simulink model "ucr_time_series_anomaly_detection_2021"  (R2021b)
settings: Solver=FixedStepDiscrete  StartTime=0.0  StopTime=100  FixedStep=0.01  RelTol=1e-3
libraries: wnnlib x38
settings Model: Creator=20214358  LastModifiedBy=20214358
settings HardwareCC: ProdLongLongMode=on  TargetBitPerPointer=64  TargetBitPerSizeT=64  TargetBitPerPtrDiffT=64  TargetLargestAtomicFloat=Float  TargetIntDivRoundTo=Zero  TargetEndianess=LittleEndian  TargetWordSize=64  TargetHWDeviceType=Intel->x86-64 (Windows64)

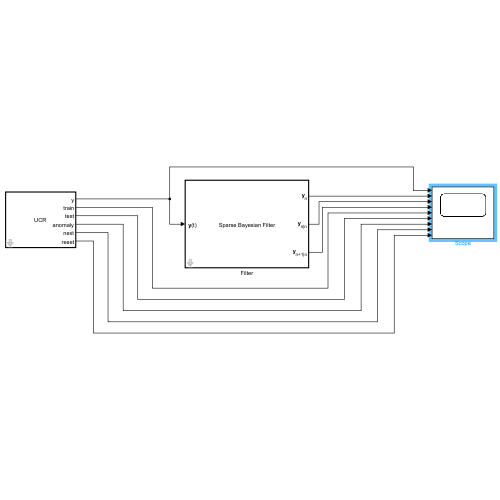
[thumbnail: Simulink's stored preview of the top-level diagram]
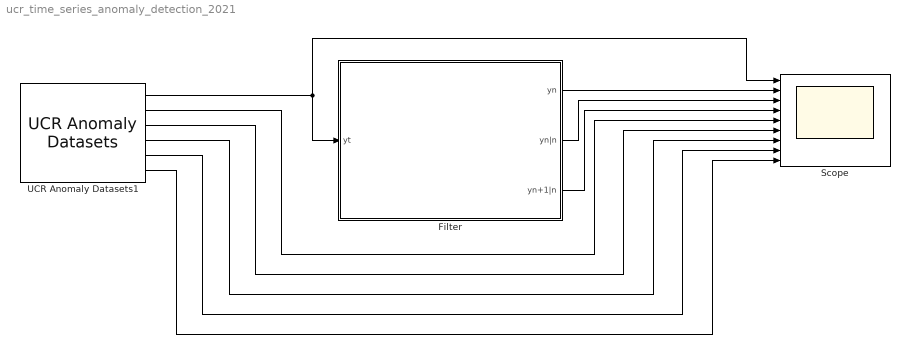
== system ucr_time_series_anomaly_detection_2021 ==
  Filter : Subsystem  TreatAsAtomicUnit=on  mask{filter_match_tolerance=1, filter_number_of_random_flips=16, sample_time=0.01, observation_dense_vector_length=1, observation_sparse_vector_length=2048, observation_memory_size=[1023 1024], observation_hamming_distance=[2 32], observation_vgram_array_length=4096, observation_number_of_samples=96, dynamics_memory_size=[1023 1024], dynamics_hamming_distance=[2 32], dynamics_vgram_array_length=2048, dynamics_number_of_samples=96, codec_number_of_sparse_vectors=4096, codec_learning_rate=0.00000000000000000000001, codec_min_bounds=[-10], codec_max_bounds=[10], codec_sparse_vectors_file='C:\Users\20214358\Workspace\wnnlib\wnndata\4k_sparse_vectors_seed_0.npz'}
      mask prompts: filter_match_tolerance "Match tolerance"; filter_number_of_random_flips "Number of random flips"; sample_time "Sample time"; observation_dense_vector_length "Dense vector length"; observation_sparse_vector_length "Sparse vector length"; observation_memory_size "Memory size"; observation_hamming_distance "Hamming distance"; observation_vgram_array_length "VGRAM array length"; observation_number_of_samples "Number of samples"; dynamics_memory_size "Memory size"; dynamics_hamming_distance "Hamming distance"; dynamics_vgram_array_length "VGRAM array length"; dynamics_number_of_samples "Number of samples"; codec_number_of_sparse_vectors "Number of sparse vectors"; codec_learning_rate "Learning rate"; codec_min_bounds "Minimum bounds"; codec_max_bounds "Maximum bounds"; codec_sparse_vectors_file "Sparse vectors file"
      mask init:
      | codec_max_kdtree_depth = ceil(log2(codec_number_of_sparse_vectors));
      | codec_min_splitting_volume = prod(codec_max_bounds - codec_min_bounds)/codec_number_of_sparse_vectors;
      | codec_sparse_vectors_file = char(codec_sparse_vectors_file);
      mask DialogControl FilterParams Prompt: Filter
      mask DialogControl ObservationModelParams Prompt: Observation model
      mask DialogControl DynamicModelParams Prompt: Dynamic model
      mask DialogControl CodecParams Prompt: Codec
      mask Display:
      | disp('Sparse Bayesian Filter','interpreter','tex');
      | port_label('input', 1,'{\bf y}(t)','interpreter','tex');
      | port_label('output', 1,'{\bf y}_{n}','interpreter','tex');
      | port_label('output', 2,'{\bf y}_{n|n}','interpreter','tex');
      | port_label('output', 3,'{\bf y}_{n+1|n}','interpreter','tex');
  Scope : Scope  NumInputPorts=9
  UCR Anomaly Datasets1 : wnnlib/Sources/UCR Anomaly Datasets  ucr_datasets_file='C:\Users\20214358\Workspace\wnnlib\wnndata\ucr_time_series_anomaly_datasets_2021.mat'  ucr_norm_flag=on  ucr_initial_dataset_idx=1  ucr_final_dataset_idx=250  ucr_sample_time=0.05
      settings: SourceProductName=Weightless Neural Networks Toolbox
  wires:
  Filter/2(yn|n) -> Scope/3
  UCR Anomaly Datasets1/1 -> Filter/1(yt), Scope/1
  Filter/1(yn) -> Scope/2
  Filter/3(yn+1|n) -> Scope/4
  UCR Anomaly Datasets1/2 -> Scope/5
  UCR Anomaly Datasets1/3 -> Scope/6
  UCR Anomaly Datasets1/4 -> Scope/7
  UCR Anomaly Datasets1/5 -> Scope/8
  UCR Anomaly Datasets1/6 -> Scope/9

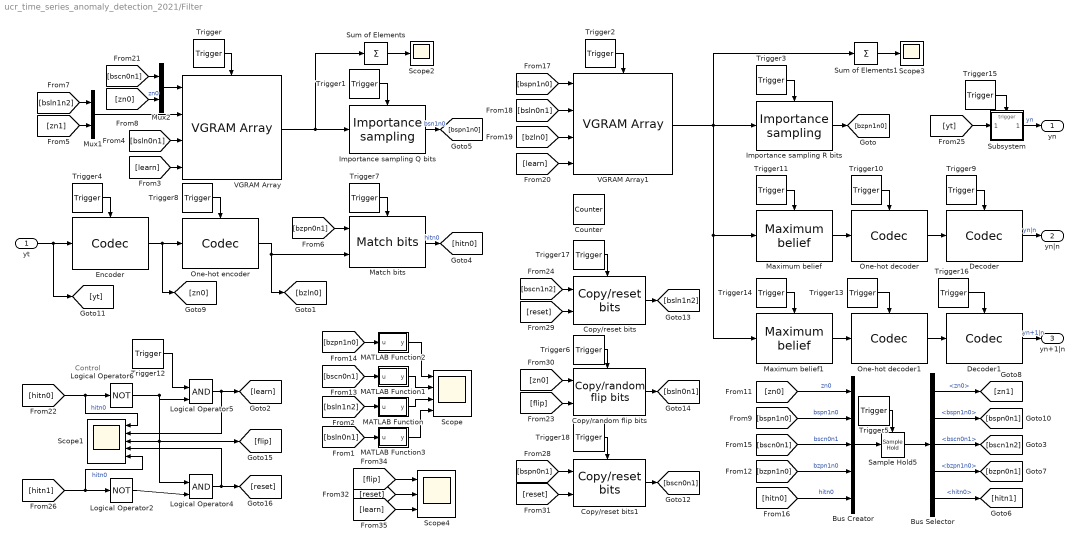
== system ucr_time_series_anomaly_detection_2021/Filter ==
  note: Control
  yt : Inport
  Bus Creator : BusCreator  Inputs=5
  Bus Selector : BusSelector  OutputSignals=zn0,bspn1n0,bscn0n1,bzpn1n0,hitn0
  Copy/random flip bits : wnnlib/Utilities/Copy//random flip bits  nNumberOfFlips=filter_number_of_random_flips
      settings: SourceProductName=Weightless Neural Networks Toolbox
  Copy/reset bits : wnnlib/Utilities/Copy//reset bits
      settings: SourceProductName=Weightless Neural Networks Toolbox
  Copy/reset bits1 : wnnlib/Utilities/Copy//reset bits
      settings: SourceProductName=Weightless Neural Networks Toolbox
  Counter : wnnlib/Sources/Counter  number_of_steps=4  sample_time=sample_time
      settings: SourceProductName=Weightless Neural Networks Toolbox
  Decoder : wnnlib/Utilities/Codec  codec_id=0  dense_vector_length=observation_dense_vector_length  sparse_vector_length=observation_sparse_vector_length  max_depth=codec_max_kdtree_depth  learning_rate=codec_learning_rate  min_splitting_volume=codec_min_splitting_volume  min_bounds=codec_min_bounds  max_bounds=codec_max_bounds  sparse_vectors_file=codec_sparse_vectors_file  debug_flag=off  codec_type=Decoder  number_of_sparse_vectors=65536
      settings: SourceProductName=Weightless Neural Networks Toolbox
  Decoder1 : wnnlib/Utilities/Codec  codec_id=0  dense_vector_length=observation_dense_vector_length  sparse_vector_length=observation_sparse_vector_length  max_depth=codec_max_kdtree_depth  learning_rate=codec_learning_rate  min_splitting_volume=codec_min_splitting_volume  min_bounds=codec_min_bounds  max_bounds=codec_max_bounds  sparse_vectors_file=codec_sparse_vectors_file  debug_flag=off  codec_type=Decoder  number_of_sparse_vectors=65536
      settings: SourceProductName=Weightless Neural Networks Toolbox
  Encoder : wnnlib/Utilities/Codec  codec_id=0  dense_vector_length=observation_dense_vector_length  sparse_vector_length=observation_sparse_vector_length  max_depth=codec_max_kdtree_depth  learning_rate=codec_learning_rate  min_splitting_volume=codec_min_splitting_volume  min_bounds=codec_min_bounds  max_bounds=codec_max_bounds  sparse_vectors_file=codec_sparse_vectors_file  debug_flag=off  codec_type=Encoder  number_of_sparse_vectors=65536
      settings: SourceProductName=Weightless Neural Networks Toolbox
  Importance sampling Q bits : wnnlib/Utilities/Importance sampling  nSamples=dynamics_number_of_samples
      settings: SourceProductName=Weightless Neural Networks Toolbox
  Importance sampling R bits : wnnlib/Utilities/Importance sampling  nSamples=observation_number_of_samples
      settings: SourceProductName=Weightless Neural Networks Toolbox
  Logical Operator2 : Logic  Operator=NOT  IconShape=distinctive  AllPortsSameDT=off  OutDataTypeStr=boolean
  Logical Operator4 : Logic  IconShape=distinctive  AllPortsSameDT=off  OutDataTypeStr=boolean
  Logical Operator5 : Logic  IconShape=distinctive  AllPortsSameDT=off  OutDataTypeStr=boolean
  Logical Operator6 : Logic  Operator=NOT  IconShape=distinctive  AllPortsSameDT=off  OutDataTypeStr=boolean
  MATLAB Function : MATLAB Function  TreatAsAtomicUnit=on
  MATLAB Function1 : MATLAB Function  TreatAsAtomicUnit=on
  MATLAB Function2 : MATLAB Function  TreatAsAtomicUnit=on
  MATLAB Function3 : MATLAB Function  TreatAsAtomicUnit=on
  Match bits : wnnlib/Utilities/Match bits  nMatchTolerance=filter_match_tolerance
      settings: SourceProductName=Weightless Neural Networks Toolbox
  Maximum belief : wnnlib/Utilities/Maximum belief  SystemSampleTime=-1  VariantActivationTime=update diagram  Latency=0  AutoFrameSizeCalculation=off
      settings: SourceProductName=Weightless Neural Networks Toolbox
  Maximum belief1 : wnnlib/Utilities/Maximum belief  SystemSampleTime=-1  VariantActivationTime=update diagram  Latency=0  AutoFrameSizeCalculation=off
      settings: SourceProductName=Weightless Neural Networks Toolbox
  Mux1 : Mux  Inputs=2
  Mux2 : Mux  Inputs=2
  One-hot decoder : wnnlib/Utilities/Codec  codec_id=0  dense_vector_length=observation_dense_vector_length  sparse_vector_length=observation_sparse_vector_length  max_depth=codec_max_kdtree_depth  learning_rate=codec_learning_rate  min_splitting_volume=codec_min_splitting_volume  min_bounds=codec_min_bounds  max_bounds=codec_max_bounds  sparse_vectors_file=codec_sparse_vectors_file  debug_flag=off  codec_type=OneHotDecoder  number_of_sparse_vectors=codec_number_of_sparse_vectors
      settings: SourceProductName=Weightless Neural Networks Toolbox
  One-hot decoder1 : wnnlib/Utilities/Codec  codec_id=0  dense_vector_length=observation_dense_vector_length  sparse_vector_length=observation_sparse_vector_length  max_depth=codec_max_kdtree_depth  learning_rate=codec_learning_rate  min_splitting_volume=codec_min_splitting_volume  min_bounds=codec_min_bounds  max_bounds=codec_max_bounds  sparse_vectors_file=codec_sparse_vectors_file  debug_flag=off  codec_type=OneHotDecoder  number_of_sparse_vectors=codec_number_of_sparse_vectors
      settings: SourceProductName=Weightless Neural Networks Toolbox
  One-hot encoder : wnnlib/Utilities/Codec  codec_id=0  dense_vector_length=observation_dense_vector_length  sparse_vector_length=observation_sparse_vector_length  max_depth=codec_max_kdtree_depth  learning_rate=codec_learning_rate  min_splitting_volume=codec_min_splitting_volume  min_bounds=codec_min_bounds  max_bounds=codec_max_bounds  sparse_vectors_file=codec_sparse_vectors_file  debug_flag=off  codec_type=OneHotEncoder  number_of_sparse_vectors=codec_number_of_sparse_vectors
      settings: SourceProductName=Weightless Neural Networks Toolbox
  Sample Hold5 : wnnlib/Utilities/Sample Hold  sample_time=-1
      settings: SourceProductName=Weightless Neural Networks Toolbox
  Scope : Scope  NumInputPorts=4
  Scope1 : Scope  NumInputPorts=5
  Scope2 : Scope
  Scope3 : Scope
  Scope4 : Scope  NumInputPorts=3
  Subsystem : Subsystem
  Sum of Elements : Sum  Inputs=+
  Sum of Elements1 : Sum  Inputs=+
  Trigger : wnnlib/Sources/Trigger  selected_steps=[0 2]
      settings: SourceProductName=Weightless Neural Networks Toolbox
  Trigger1 : wnnlib/Sources/Trigger  selected_steps=[0 2]
      settings: SourceProductName=Weightless Neural Networks Toolbox
  Trigger{4,6..12,15,17..18} (11 alike) : wnnlib/Sources/Trigger  selected_steps=0
      settings: SourceProductName=Weightless Neural Networks Toolbox
  Trigger{3,13..14,16} (4 alike) : wnnlib/Sources/Trigger  selected_steps=2
      settings: SourceProductName=Weightless Neural Networks Toolbox
  Trigger2 : wnnlib/Sources/Trigger  selected_steps=[0 2]
      settings: SourceProductName=Weightless Neural Networks Toolbox
  Trigger5 : wnnlib/Sources/Trigger  selected_steps=4
      settings: SourceProductName=Weightless Neural Networks Toolbox
  VGRAM Array : wnnlib/Models/VGRAM Array  array_id=0  min_mem_size=dynamics_memory_size(1)  max_mem_size=dynamics_memory_size(2)  min_dist=dynamics_hamming_distance(1)  max_dist=dynamics_hamming_distance(2)  pattern_length=dynamics_vgram_array_length+observation_sparse_vector_length  output_dims=[dynamics_vgram_array_length 1]  debug_flag=off
      settings: SourceProductName=Weightless Neural Networks Toolbox
  VGRAM Array1 : wnnlib/Models/VGRAM Array  array_id=1  min_mem_size=observation_memory_size(1)  max_mem_size=observation_memory_size(2)  min_dist=observation_hamming_distance(1)  max_dist=observation_hamming_distance(2)  pattern_length=dynamics_vgram_array_length  output_dims=[observation_vgram_array_length 1]  debug_flag=off
      settings: SourceProductName=Weightless Neural Networks Toolbox
  yn : Outport
  yn|n : Outport  Port=2
  yn+1|n : Outport  Port=3
  wires:
  Trigger1/1 -> Importance sampling Q bits/Trigger
  Trigger2/1 -> VGRAM Array1/Trigger
  VGRAM Array/1 -> Sum of Elements/1, Importance sampling Q bits/1
  Trigger4/1 -> Encoder/Trigger
  Trigger7/1 -> Match bits/Trigger
  Trigger6/1 -> Copy/random flip bits/Trigger
  Trigger/1 -> VGRAM Array/Trigger
  Trigger3/1 -> Importance sampling R bits/Trigger
  [bzpn0n1] -> Match bits/1
  Trigger8/1 -> One-hot encoder/Trigger
  [bsln0n1] -> VGRAM Array1/2
  Decoder/1 -> yn|n/1  "yn|n"
  Trigger9/1 -> Decoder/Trigger
  One-hot decoder/1 -> Decoder/1
  Trigger10/1 -> One-hot decoder/Trigger
  Trigger11/1 -> Maximum belief/Trigger
  [learn] -> VGRAM Array1/4
  [learn] -> VGRAM Array/4
  yt/1 -> [yt], Encoder/1
  Encoder/1 -> [zn0], One-hot encoder/1
  [bscn0n1] -> Mux2/1
  Mux1/1 -> VGRAM Array/2
  [bsln1n2] -> Mux1/1
  Maximum belief/1 -> One-hot decoder/1
  Mux2/1 -> VGRAM Array/1
  [zn0] -> Mux2/2  "zn0"
  Importance sampling Q bits/1 -> [bspn1n0]  "bsn1n0"
  One-hot encoder/1 -> Match bits/2, [bzln0]
  [bsln0n1] -> VGRAM Array/3
  [bzln0] -> VGRAM Array1/3
  Trigger15/1 -> Subsystem/Trigger
  Subsystem/1(Out1) -> yn/1  "yn"
  Decoder1/1 -> yn+1|n/1  "yn+1|n"
  One-hot decoder1/1 -> Decoder1/1
  Maximum belief1/1 -> One-hot decoder1/1
  Trigger14/1 -> Maximum belief1/Trigger
  Trigger13/1 -> One-hot decoder1/Trigger
  Trigger16/1 -> Decoder1/Trigger
  [hitn1] -> Scope1/5, Logical Operator2/1  "hitn0"
  Logical Operator5/1 -> Scope1/2, [learn]
  Logical Operator2/1 -> Logical Operator4/2
  Match bits/1 -> [hitn0]  "hitn0"
  [yt] -> Subsystem/1(In1)
  [bsln1n2] -> MATLAB Function/1(u)
  MATLAB Function1/1(y) -> Scope/2
  MATLAB Function2/1(y) -> Scope/1
  MATLAB Function/1(y) -> Scope/3
  [bscn0n1] -> MATLAB Function1/1(u)
  Trigger5/1 -> Sample Hold5/Trigger
  [hitn0] -> Bus Creator/5  "hitn0"
  Bus Selector/1 -> [zn1]  "<zn0>"
  Bus Creator/1 -> Sample Hold5/1
  Bus Selector/5 -> [hitn1]  "<hitn0>"
  [zn0] -> Bus Creator/1  "zn0"
  Bus Selector/4 -> [bzpn0n1]  "<bzpn1n0>"
  [bspn1n0] -> Bus Creator/2  "bspn1n0"
  MATLAB Function3/1(y) -> Scope/4
  Sample Hold5/1 -> Bus Selector/1
  [bscn0n1] -> Bus Creator/3  "bscn0n1"
  [bzpn1n0] -> Bus Creator/4  "bzpn1n0"
  Bus Selector/2 -> [bspn0n1]  "<bspn1n0>"
  [bzpn1n0] -> MATLAB Function2/1(u)
  Bus Selector/3 -> [bscn1n2]  "<bscn0n1>"
  Copy/reset bits/1 -> [bsln1n2]
  Trigger12/1 -> Logical Operator5/1
  Logical Operator6/1 -> [flip], Logical Operator4/1, Scope1/3, Logical Operator5/2
  Logical Operator4/1 -> Scope1/4, [reset]
  [flip] -> Copy/random flip bits/2
  [reset] -> Copy/reset bits/2
  [bsln0n1] -> MATLAB Function3/1(u)
  Importance sampling R bits/1 -> [bzpn1n0]
  Sum of Elements/1 -> Scope2/1
  [bspn1n0] -> VGRAM Array1/1
  [hitn0] -> Scope1/1, Logical Operator6/1  "hitn0"
  Sum of Elements1/1 -> Scope3/1
  VGRAM Array1/1 -> Sum of Elements1/1, Maximum belief1/1, Maximum belief/1, Importance sampling R bits/1
  [bscn1n2] -> Copy/reset bits/1
  [zn1] -> Mux1/2
  [reset] -> Scope4/2
  [flip] -> Scope4/1
  [learn] -> Scope4/3
  Trigger17/1 -> Copy/reset bits/Trigger
  Trigger18/1 -> Copy/reset bits1/Trigger
  Copy/reset bits1/1 -> [bscn0n1]
  [reset] -> Copy/reset bits1/2
  [zn0] -> Copy/random flip bits/1
  Copy/random flip bits/1 -> [bsln0n1]
  [bspn0n1] -> Copy/reset bits1/1

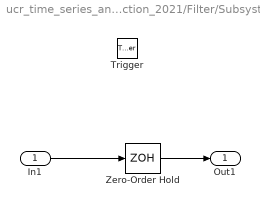
== system ucr_time_series_anomaly_detection_2021/Filter/Subsystem ==
  In1 : Inport
  Trigger : TriggerPort  VariantControl=(inherit)  PortDimensions=1
  Zero-Order Hold : ZeroOrderHold  SampleTime=-1
  Out1 : Outport
  wires:
  Zero-Order Hold/1 -> Out1/1
  In1/1 -> Zero-Order Hold/1

== matlab function ucr_time_series_anomaly_detection_2021/Filter/MATLAB Function ==
  data: u input; y output
function y = fcn(u)
y=0;
for i=1:length(u)
    if u(i) ~= 0
        y = y+i;
    end
end

== matlab function ucr_time_series_anomaly_detection_2021/Filter/MATLAB Function2 ==
  data: u input; y output
function y = fcn(u)
y=0;
for i=1:length(u)
    if u(i) ~= 0
        y = y+i;
    end
end

== matlab function ucr_time_series_anomaly_detection_2021/Filter/MATLAB Function3 ==
  data: u input; y output
function y = fcn(u)
y=0;
for i=1:length(u)
    if u(i) ~= 0
        y = y+i;
    end
end

== matlab function ucr_time_series_anomaly_detection_2021/Filter/MATLAB Function1 ==
  data: u input; y output
function y = fcn(u)
y=0;
for i=1:length(u)
    if u(i) ~= 0
        y = y+i;
    end
end
